simulink model "gm_sampleModel2081_5_sub"  (R2023a)
settings: Solver=VariableStepAuto  StartTime=0.0  StopTime=10.0  RelTol=1e-3
libraries: hdlsllib x3, simulink x3
settings Model: Creator=user1  LastModifiedBy=user1
settings OptimizationCC: BlockReduction=off  ConditionallyExecuteInputs=off
settings DebuggingCC: InheritedTsInSrcMsg=none

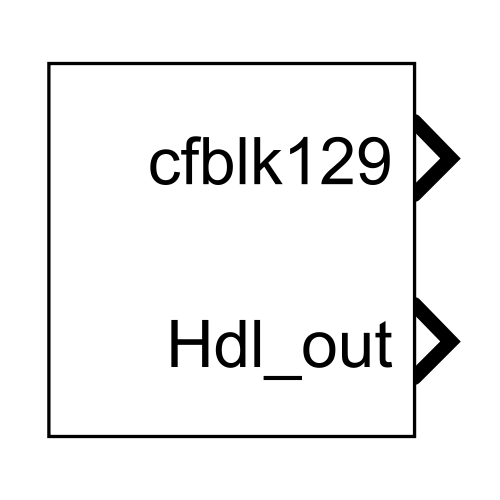
[thumbnail: Simulink's stored preview of the top-level diagram]
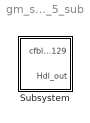
== system gm_sampleModel2081_5_sub ==
  Subsystem : Subsystem

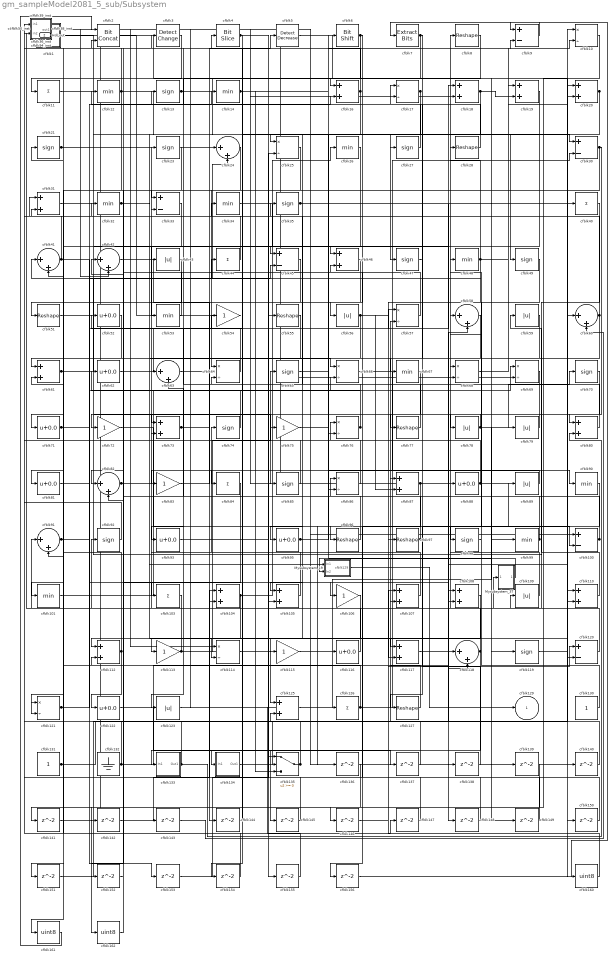
== system gm_sampleModel2081_5_sub/Subsystem ==
  Mysubsystem_19 : Subsystem
  Mysubsystem_37 : Subsystem
  cfblk1 : Subsystem  mask(Compare To Zero){relop=<=, OutDataTypeStr=uint8, ZeroCross=on}
      mask prompts: relop "Simulink:masks:Operator_MP"; OutDataTypeStr "Simulink:masks:OutputDataType_MP"; ZeroCross "Simulink:masks:EnableZerocrossingDetection_MP"
      mask help: Simulink:masks:CompareToZero_MD
      mask init:
      | OutDataTypeStr = 'uint8';
      | ZeroCross = 'on';
      | blkName = 'sampleModel2081_5_sub/Subsystem/cfblk1';
      | relop = '<=';
      | setValue = 'fixdt(0, 8)';
      mask TypeOptions relop: == | ~= | < | <= | >= | >
      mask TypeOptions OutDataTypeStr: Simulink:masks:uint8 | Simulink:masks:boolean
      mask Callback ZeroCross: sl('zeroCrossEnable', gcbh);
      mask Display: disp([relop,' 0'])
  cfblk{10,17,25,57,64,66,68..69,76,86,114,121} (12 alike) : Product  Inputs=*/  OutDataTypeStr=uint8  RndMeth=Zero  SaturateOnIntegerOverflow=on
  cfblk{9,30,33,45,100,120} (6 alike) : Sum  Inputs=+-  OutDataTypeStr=uint8
  cfblk{12,14,26,32,34,48,53,67,90,99,101} (11 alike) : MinMax  OutDataTypeStr=uint8
  cfblk{11,40,44,84,103,126} (6 alike) : Sum  Inputs=+  OutDataTypeStr=uint8
  cfblk{16,18..20,31,46,61,73,80,87,104..105,107..108,110,112,117,125} (18 alike) : Sum  OutDataTypeStr=uint8
  cfblk{54,72,75,83,106,113,115} (7 alike) : Gain  OutDataTypeStr=uint8
  cfblk{43,56,59,78..79,89,109,123} (8 alike) : Abs  OutDataTypeStr=uint8  SaturateOnIntegerOverflow=off
  cfblk111_inst : Subsystem
  cfblk{52,62,71,81,88,93,95,116,122} (9 alike) : Bias  Bias=0.0  SaturateOnIntegerOverflow=off
  cfblk{24,41..42,58,60,63,82,91,118} (9 alike) : Sum  Inputs=|++  OutDataTypeStr=uint8
  cfblk{13,21,23,27,35,47,49,65,70,74,85,92,98,119} (14 alike) : Signum
  cfblk124_inst : Subsystem
  cfblk{8,28,51,55,77,96..97,127} (8 alike) : Reshape
  cfblk130 : Constant  OutDataTypeStr=uint8  SampleTime=-1
  cfblk131 : Constant  OutDataTypeStr=uint8  SampleTime=-1
  cfblk132 : Ground
  cfblk133 : Subsystem
  cfblk134 : Subsystem
  cfblk135 : Switch  OutDataTypeStr=uint8  SaturateOnIntegerOverflow=off  InputSameDT=off
  cfblk{136..156} (21 alike) : Delay  SampleTime=1
  cfblk15_inst : Subsystem
  cfblk160 : DataTypeConversion  OutDataTypeStr=uint8  SaturateOnIntegerOverflow=off  RndMeth=Floor
  cfblk161 : DataTypeConversion  OutDataTypeStr=uint8  SaturateOnIntegerOverflow=off  RndMeth=Floor
  cfblk162 : DataTypeConversion  OutDataTypeStr=uint8  SaturateOnIntegerOverflow=off  RndMeth=Floor
  cfblk2 : hdlsllib/Logic and Bit Operations/Bit Concat  numInputs=2
  cfblk3 : simulink/Logic and Bit Operations/Detect Change  vinit=0  OutDataTypeStr=uint8
      settings: LibrarySourceBlock=|
      | hdlsllib/Logic and Bit
      | Operations/Detect
      | Change
  cfblk36_inst : Subsystem
  cfblk38_inst : Subsystem
  cfblk39_inst : Subsystem
  cfblk4 : hdlsllib/Logic and Bit Operations/Bit Slice  lidx=7  ridx=0
  cfblk5 : simulink/Logic and Bit Operations/Detect Decrease  vinit=0.0  OutDataTypeStr=uint8
      settings: LibrarySourceBlock=|
      | hdlsllib/Logic and Bit
      | Operations/Detect
      | Decrease
  cfblk50_inst : Subsystem
  cfblk6 : hdlsllib/Logic and Bit Operations/Bit Shift  mode=Shift Left Logical  N=0
  cfblk7 : simulink/Logic and Bit Operations/Extract Bits  bitsToExtract=Upper half  numBits=8  bitIdxRange=[0 7]  outScalingMode=Preserve fixed-point scaling
      settings: LibrarySourceBlock=|
      | hdlsllib/Logic and Bit
      | Operations/Extract Bits
  cfblk94_inst : Subsystem
  cfblk129 : Outport  OutDataTypeStr=uint8  SampleTime=1  VectorParamsAs1DForOutWhenUnconnected=off
  Hdl_out : Outport  Port=2  OutDataTypeStr=uint8  SampleTime=1
  wires:
  Mysubsystem_19/1(cfblk129) -> cfblk129/1
  Mysubsystem_37/1(Out1) -> Mysubsystem_19/2(In2)
  cfblk1/1(y) -> Mysubsystem_37/1(In1)
  cfblk10/1 -> cfblk146/1
  cfblk100/1 -> cfblk63/2, cfblk42/1
  cfblk101/1 -> cfblk69/1
  cfblk103/1 -> cfblk38_inst/2(in2)
  cfblk104/1 -> cfblk113/1, cfblk26/1
  cfblk105/1 -> cfblk74/1
  cfblk106/1 -> cfblk125/1
  cfblk107/1 -> cfblk23/1
  cfblk108/1 -> cfblk112/1
  cfblk109/1 -> cfblk8/1
  cfblk11/1 -> cfblk30/1
  cfblk110/1 -> cfblk59/1
  cfblk111_inst/1(out1) -> cfblk24/1, Hdl_out/1, cfblk40/1
  cfblk112/1 -> cfblk39_inst/2(in2), cfblk122/1
  cfblk113/1 -> cfblk91/1, cfblk65/1
  cfblk114/1 -> cfblk55/1
  cfblk115/1 -> cfblk99/1
  cfblk116/1 -> cfblk92/1
  cfblk117/1 -> cfblk118/1
  cfblk118/1 -> cfblk33/2, cfblk76/1, cfblk145/1
  cfblk119/1 -> cfblk20/2
  cfblk12/1 -> cfblk36_inst/1(in1), cfblk110/1, cfblk141/1
  cfblk120/1 -> cfblk68/1
  cfblk121/1 -> cfblk13/1, cfblk66/2
  cfblk122/1 -> cfblk134/1(In1)
  cfblk123/1 -> cfblk147/1
  cfblk124_inst/1(out1) -> cfblk111_inst/1(in1)
  cfblk125/1 -> cfblk79/1
  cfblk126/1 -> cfblk41/2, cfblk30/2
  cfblk127/1 -> cfblk57/2
  cfblk13/1 -> cfblk47/1, cfblk16/2, cfblk16/1
  cfblk130/1 -> cfblk41/1
  cfblk131/1 -> cfblk87/1, cfblk10/1
  cfblk132/1 -> cfblk94_inst/1(in1), cfblk68/2
  cfblk133/1(Out1) -> cfblk80/2, cfblk36_inst/2(in2)
  cfblk134/1(Out1) -> cfblk60/1
  cfblk135/1 -> cfblk21/1, cfblk133/1(In1)
  cfblk136/1 -> cfblk162/1
  cfblk137/1 -> cfblk38_inst/1(in1)
  cfblk138/1 -> cfblk17/1
  cfblk139/1 -> cfblk161/1
  cfblk14/1 -> cfblk9/2, cfblk135/3
  cfblk140/1 -> cfblk107/2
  cfblk141/1 -> cfblk58/2
  cfblk142/1 -> cfblk104/1
  cfblk143/1 -> cfblk60/2
  cfblk144/1 -> cfblk64/2
  cfblk145/1 -> cfblk61/2
  cfblk146/1 -> cfblk120/1
  cfblk147/1 -> cfblk124_inst/2(in2)
  cfblk148/1 -> cfblk86/1
  cfblk149/1 -> cfblk112/2
  cfblk15_inst/1(out1) -> cfblk89/1
  cfblk150/1 -> cfblk135/2
  cfblk151/1 -> cfblk125/2
  cfblk152/1 -> cfblk82/2
  cfblk153/1 -> cfblk25/2
  cfblk154/1 -> cfblk91/2
  cfblk155/1 -> cfblk111_inst/2(in2)
  cfblk156/1 -> cfblk9/1
  cfblk16/1 -> cfblk39_inst/1(in1), cfblk114/2
  cfblk160/1 -> cfblk107/1
  cfblk161/1 -> cfblk2/1
  cfblk162/1 -> cfblk2/2
  cfblk17/1 -> cfblk95/1, cfblk86/2
  cfblk18/1 -> cfblk19/2, cfblk25/1
  cfblk19/1 -> cfblk76/2
  cfblk2/1 -> cfblk160/1
  cfblk20/1 -> cfblk49/1, cfblk45/1
  cfblk21/1 -> cfblk27/1, cfblk106/1
  cfblk23/1 -> cfblk81/1
  cfblk24/1 -> cfblk51/1
  cfblk25/1 -> cfblk64/1
  cfblk26/1 -> cfblk121/2
  cfblk27/1 -> cfblk3/1
  cfblk28/1 -> cfblk12/1
  cfblk3/1 -> cfblk11/1
  cfblk30/1 -> cfblk80/1, cfblk72/1
  cfblk31/1 -> cfblk46/1
  cfblk32/1 -> cfblk117/1, cfblk66/1, Mysubsystem_19/1(In1)
  cfblk33/1 -> cfblk53/1
  cfblk34/1 -> cfblk138/1
  cfblk35/1 -> cfblk149/1, cfblk148/1
  cfblk36_inst/1(out1) -> cfblk116/1, cfblk140/1
  cfblk38_inst/1(out1) -> cfblk88/1, cfblk18/2
  cfblk39_inst/1(out1) -> cfblk42/2, cfblk69/2, cfblk126/1
  cfblk4/1 -> cfblk155/1, cfblk154/1
  cfblk40/1 -> cfblk109/1
  cfblk41/1 -> cfblk15_inst/1(in1), cfblk153/1
  cfblk42/1 -> cfblk144/1
  cfblk43/1 -> cfblk61/1
  cfblk44/1 -> cfblk50_inst/1(in1)
  cfblk45/1 -> cfblk123/1
  cfblk46/1 -> cfblk73/1
  cfblk47/1 -> cfblk17/2
  cfblk48/1 -> cfblk28/1, cfblk117/2, cfblk10/2
  cfblk49/1 -> cfblk98/1
  cfblk5/1 -> cfblk139/1
  cfblk50_inst/1(out1) -> cfblk114/1
  cfblk51/1 -> cfblk135/1
  cfblk52/1 -> cfblk151/1
  cfblk53/1 -> cfblk94_inst/2(in2)
  cfblk54/1 -> cfblk1/1(u)
  cfblk55/1 -> cfblk93/1
  cfblk56/1 -> cfblk97/1, cfblk87/2, cfblk71/1, cfblk105/1
  cfblk57/1 -> cfblk43/1
  cfblk58/1 -> cfblk82/1
  cfblk59/1 -> cfblk84/1
  cfblk6/1 -> cfblk56/1, cfblk33/1
  cfblk60/1 -> cfblk31/2, cfblk19/1, cfblk101/1
  cfblk61/1 -> cfblk24/2, cfblk44/1
  cfblk62/1 -> cfblk18/1
  cfblk63/1 -> cfblk137/1
  cfblk64/1 -> cfblk32/1
  cfblk65/1 -> cfblk119/1
  cfblk66/1 -> cfblk108/1
  cfblk67/1 -> cfblk115/1
  cfblk68/1 -> cfblk20/1
  cfblk69/1 -> cfblk85/1
  cfblk7/1 -> cfblk105/2, cfblk67/1
  cfblk70/1 -> cfblk152/1
  cfblk71/1 -> cfblk45/2, cfblk57/1
  cfblk72/1 -> cfblk150/1
  cfblk73/1 -> cfblk96/1, cfblk75/1
  cfblk74/1 -> cfblk62/1
  cfblk75/1 -> cfblk90/1
  cfblk76/1 -> cfblk63/1, cfblk54/1
  cfblk77/1 -> cfblk52/1
  cfblk78/1 -> cfblk77/1, cfblk70/1
  cfblk79/1 -> cfblk78/1
  cfblk8/1 -> cfblk103/1
  cfblk80/1 -> cfblk35/1
  cfblk81/1 -> cfblk14/1
  cfblk82/1 -> cfblk104/2, cfblk136/1
  cfblk83/1 -> cfblk5/1
  cfblk84/1 -> cfblk142/1
  cfblk85/1 -> cfblk34/1
  cfblk86/1 -> cfblk124_inst/1(in1)
  cfblk87/1 -> cfblk110/2, cfblk156/1
  cfblk88/1 -> cfblk4/1, cfblk100/2
  cfblk89/1 -> cfblk83/1
  cfblk9/1 -> cfblk7/1
  cfblk90/1 -> cfblk127/1
  cfblk91/1 -> cfblk108/2, cfblk121/1
  cfblk92/1 -> cfblk15_inst/2(in2)
  cfblk93/1 -> cfblk120/2
  cfblk94_inst/1(out1) -> cfblk100/1, cfblk143/1
  cfblk95/1 -> cfblk6/1, cfblk118/2
  cfblk96/1 -> cfblk50_inst/2(in2)
  cfblk97/1 -> cfblk46/2, cfblk31/1
  cfblk98/1 -> cfblk48/1
  cfblk99/1 -> cfblk73/2, cfblk58/1

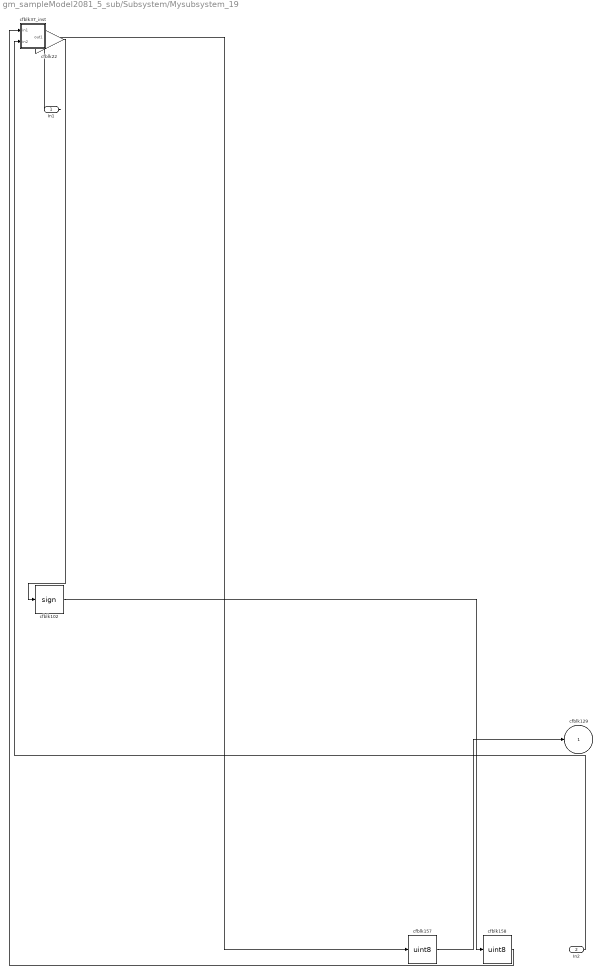
== system gm_sampleModel2081_5_sub/Subsystem/Mysubsystem_19 ==
  In1 : Inport  OutDataTypeStr=uint8  PortDimensions=1  SampleTime=1
  In2 : Inport  Port=2  OutDataTypeStr=uint8  PortDimensions=1  SampleTime=1
  cfblk102 : Signum
  cfblk157 : DataTypeConversion  OutDataTypeStr=uint8  SaturateOnIntegerOverflow=off  RndMeth=Floor
  cfblk158 : DataTypeConversion  OutDataTypeStr=uint8  SaturateOnIntegerOverflow=off  RndMeth=Floor
  cfblk22 : Gain
  cfblk37_inst : Subsystem
  cfblk129 : Outport  SampleTime=1  VectorParamsAs1DForOutWhenUnconnected=off
  wires:
  In1/1 -> cfblk22/1
  In2/1 -> cfblk37_inst/2(in2)
  cfblk102/1 -> cfblk158/1
  cfblk157/1 -> cfblk129/1
  cfblk158/1 -> cfblk37_inst/1(in1)
  cfblk22/1 -> cfblk102/1
  cfblk37_inst/1(out1) -> cfblk157/1

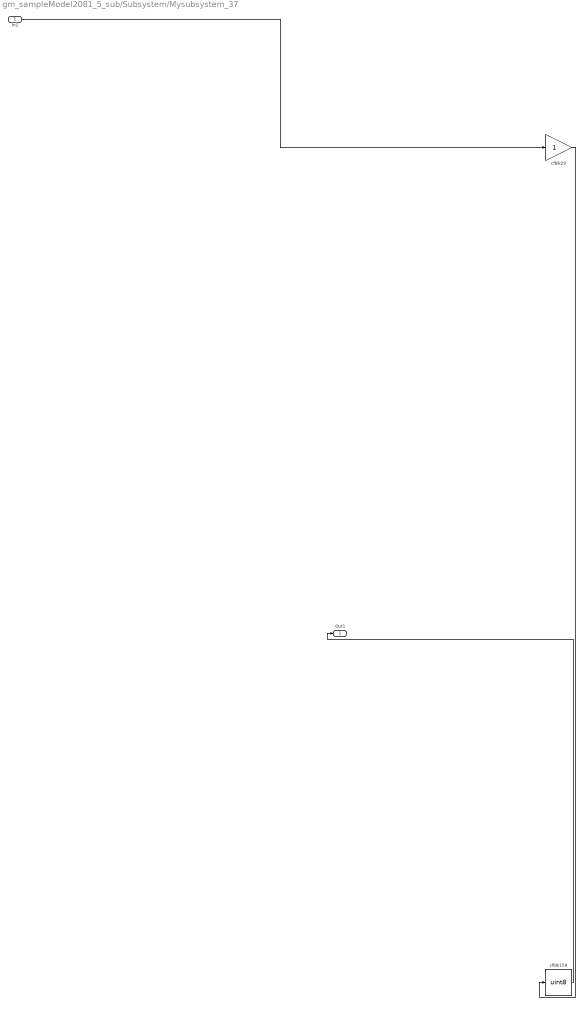
== system gm_sampleModel2081_5_sub/Subsystem/Mysubsystem_37 ==
  In1 : Inport  OutDataTypeStr=uint8  PortDimensions=1  SampleTime=1
  cfblk159 : DataTypeConversion  OutDataTypeStr=uint8  SaturateOnIntegerOverflow=off  RndMeth=Floor
  cfblk29 : Gain
  Out1 : Outport  SampleTime=1
  wires:
  In1/1 -> cfblk29/1
  cfblk159/1 -> Out1/1
  cfblk29/1 -> cfblk159/1

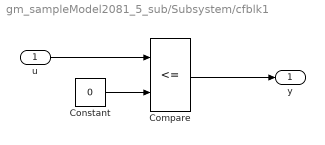
== system gm_sampleModel2081_5_sub/Subsystem/cfblk1 ==
  u : Inport  OutDataTypeStr=uint8  SampleTime=1
  Compare : RelationalOperator  Operator=<=  OutDataTypeStr=fixdt(0, 8)
  Constant : Constant  DisableCoverage=on  Value=0  OutDataTypeStr=Inherit: Inherit via back propagation  SampleTime=-1  PreserveConstantTs=on
  y : Outport  SampleTime=1
  wires:
  u/1 -> Compare/1
  Compare/1 -> y/1
  Constant/1 -> Compare/2

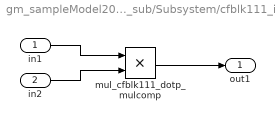
== system gm_sampleModel2081_5_sub/Subsystem/cfblk111_inst ==
  in1 : Inport  OutDataTypeStr=uint8  SampleTime=1
  in2 : Inport  Port=2  OutDataTypeStr=uint8  SampleTime=1
  mul_cfblk111_dotp_mulcomp : Product  Inputs=**  OutDataTypeStr=uint8  SampleTime=1
  out1 : Outport  OutDataTypeStr=uint8  SampleTime=1
  wires:
  in1/1 -> mul_cfblk111_dotp_mulcomp/1
  in2/1 -> mul_cfblk111_dotp_mulcomp/2
  mul_cfblk111_dotp_mulcomp/1 -> out1/1

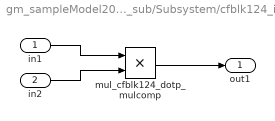
== system gm_sampleModel2081_5_sub/Subsystem/cfblk124_inst ==
  in1 : Inport  OutDataTypeStr=uint8  SampleTime=1
  in2 : Inport  Port=2  OutDataTypeStr=uint8  SampleTime=1
  mul_cfblk124_dotp_mulcomp : Product  Inputs=**  OutDataTypeStr=uint8  SampleTime=1
  out1 : Outport  OutDataTypeStr=uint8  SampleTime=1
  wires:
  in1/1 -> mul_cfblk124_dotp_mulcomp/1
  in2/1 -> mul_cfblk124_dotp_mulcomp/2
  mul_cfblk124_dotp_mulcomp/1 -> out1/1

== system gm_sampleModel2081_5_sub/Subsystem/cfblk133 ==
  In1 : Inport  OutDataTypeStr=uint8  PortDimensions=1  SampleTime=1
  Out1 : Outport  SampleTime=1
  wires:
  In1/1 -> Out1/1

== system gm_sampleModel2081_5_sub/Subsystem/cfblk134 ==
  In1 : Inport  OutDataTypeStr=uint8  PortDimensions=1  SampleTime=1
  Out1 : Outport  SampleTime=1
  wires:
  In1/1 -> Out1/1

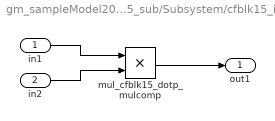
== system gm_sampleModel2081_5_sub/Subsystem/cfblk15_inst ==
  in1 : Inport  OutDataTypeStr=uint8  SampleTime=1
  in2 : Inport  Port=2  OutDataTypeStr=uint8  SampleTime=1
  mul_cfblk15_dotp_mulcomp : Product  Inputs=**  OutDataTypeStr=uint8  SampleTime=1
  out1 : Outport  OutDataTypeStr=uint8  SampleTime=1
  wires:
  in1/1 -> mul_cfblk15_dotp_mulcomp/1
  in2/1 -> mul_cfblk15_dotp_mulcomp/2
  mul_cfblk15_dotp_mulcomp/1 -> out1/1

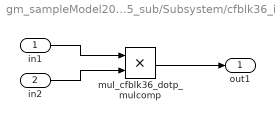
== system gm_sampleModel2081_5_sub/Subsystem/cfblk36_inst ==
  in1 : Inport  OutDataTypeStr=uint8  SampleTime=1
  in2 : Inport  Port=2  OutDataTypeStr=uint8  SampleTime=1
  mul_cfblk36_dotp_mulcomp : Product  Inputs=**  OutDataTypeStr=uint8  SampleTime=1
  out1 : Outport  OutDataTypeStr=uint8  SampleTime=1
  wires:
  in1/1 -> mul_cfblk36_dotp_mulcomp/1
  in2/1 -> mul_cfblk36_dotp_mulcomp/2
  mul_cfblk36_dotp_mulcomp/1 -> out1/1

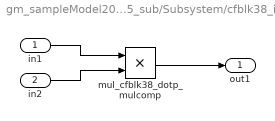
== system gm_sampleModel2081_5_sub/Subsystem/cfblk38_inst ==
  in1 : Inport  OutDataTypeStr=uint8  SampleTime=1
  in2 : Inport  Port=2  OutDataTypeStr=uint8  SampleTime=1
  mul_cfblk38_dotp_mulcomp : Product  Inputs=**  OutDataTypeStr=uint8  SampleTime=1
  out1 : Outport  OutDataTypeStr=uint8  SampleTime=1
  wires:
  in1/1 -> mul_cfblk38_dotp_mulcomp/1
  in2/1 -> mul_cfblk38_dotp_mulcomp/2
  mul_cfblk38_dotp_mulcomp/1 -> out1/1

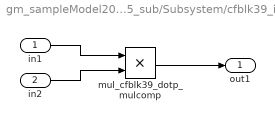
== system gm_sampleModel2081_5_sub/Subsystem/cfblk39_inst ==
  in1 : Inport  OutDataTypeStr=uint8  SampleTime=1
  in2 : Inport  Port=2  OutDataTypeStr=uint8  SampleTime=1
  mul_cfblk39_dotp_mulcomp : Product  Inputs=**  OutDataTypeStr=uint8  SampleTime=1
  out1 : Outport  OutDataTypeStr=uint8  SampleTime=1
  wires:
  in1/1 -> mul_cfblk39_dotp_mulcomp/1
  in2/1 -> mul_cfblk39_dotp_mulcomp/2
  mul_cfblk39_dotp_mulcomp/1 -> out1/1

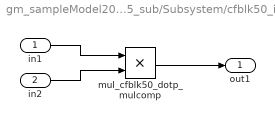
== system gm_sampleModel2081_5_sub/Subsystem/cfblk50_inst ==
  in1 : Inport  OutDataTypeStr=uint8  SampleTime=1
  in2 : Inport  Port=2  OutDataTypeStr=uint8  SampleTime=1
  mul_cfblk50_dotp_mulcomp : Product  Inputs=**  OutDataTypeStr=uint8  SampleTime=1
  out1 : Outport  OutDataTypeStr=uint8  SampleTime=1
  wires:
  in1/1 -> mul_cfblk50_dotp_mulcomp/1
  in2/1 -> mul_cfblk50_dotp_mulcomp/2
  mul_cfblk50_dotp_mulcomp/1 -> out1/1

== system gm_sampleModel2081_5_sub/Subsystem/cfblk94_inst ==
  in1 : Inport  OutDataTypeStr=uint8  SampleTime=1
  in2 : Inport  Port=2  OutDataTypeStr=uint8  SampleTime=1
  mul_cfblk94_dotp_mulcomp : Product  Inputs=**  OutDataTypeStr=uint8  SampleTime=1
  out1 : Outport  OutDataTypeStr=uint8  SampleTime=1
  wires:
  in1/1 -> mul_cfblk94_dotp_mulcomp/1
  in2/1 -> mul_cfblk94_dotp_mulcomp/2
  mul_cfblk94_dotp_mulcomp/1 -> out1/1

== system gm_sampleModel2081_5_sub/Subsystem/Mysubsystem_19/cfblk37_inst ==
  in1 : Inport  OutDataTypeStr=uint8  SampleTime=1
  in2 : Inport  Port=2  OutDataTypeStr=uint8  SampleTime=1
  mul_cfblk37_dotp_mulcomp : Product  Inputs=**  OutDataTypeStr=uint16  SampleTime=1
  out1 : Outport  OutDataTypeStr=uint16  SampleTime=1
  wires:
  in1/1 -> mul_cfblk37_dotp_mulcomp/1
  in2/1 -> mul_cfblk37_dotp_mulcomp/2
  mul_cfblk37_dotp_mulcomp/1 -> out1/1
